simulink model "NetworkModelSimpleIntersectionOptimalControl"  (R2018b)
settings: Solver=VariableStepAuto  StartTime=tStart  StopTime=tFinal  FixedStep=0.001  RelTol=1e-3
values from neighbouring files (symbols this model uses):
  Ax = [0 1  0   0 ... (first row only)    [DroneSubsystemModelling.m]
  Ay = [0 1  0   0 ... (first row only)    [DroneSubsystemModelling.m]
  Bx = [0;0;0;b1]    [DroneSubsystemModelling.m]
  By = [0;0;0;b2]    [DroneSubsystemModelling.m]
  ConflictDrone2andDrone4 = ControlDetectionFunction(tout,PositionXDrone2, PositionYDrone2, PositionXDrone4, PositionYDrone4, ConflictDrone2andDrone4)    [ConflictDetection.m]    (also in ConflictDetectionTEST.m = ControlDetectionFunction(tout,PositionXDrone2TEST, PositionY)
  Cpx = [1 0 0 0]    [DroneSubsystemModelling.m]
  Cpy = [1 0 0 0]    [DroneSubsystemModelling.m]
  Cvx = [0 1 0 0]    [DroneSubsystemModelling.m]
  Cvy = [0 1 0 0]    [DroneSubsystemModelling.m]
  theta2 = -3*180/4    (= -135)    [MotionModelling.m]
  theta4 = -180/4    (= -45)    [MotionModelling.m]
  VelocityStarX2 = vx20    [MotionModelling.m]
  VelocityStarX4 = vx40    [MotionModelling.m]
  VelocityStarY2 = vy20    [MotionModelling.m]
  VelocityStarY4 = vy40    [MotionModelling.m]
  X20 = [x20 vx20 0 0]'    [MotionModelling.m]
  X40 = [x40 vx40 0 0]'    [MotionModelling.m]
  Y20 = [y20 vy20 0 0]'    [MotionModelling.m]
  Y40 = [y40 vy40 0 0]'    [MotionModelling.m]
libraries: simulink x8
settings Model: Creator=CowUser  LastModifiedBy=CowUser

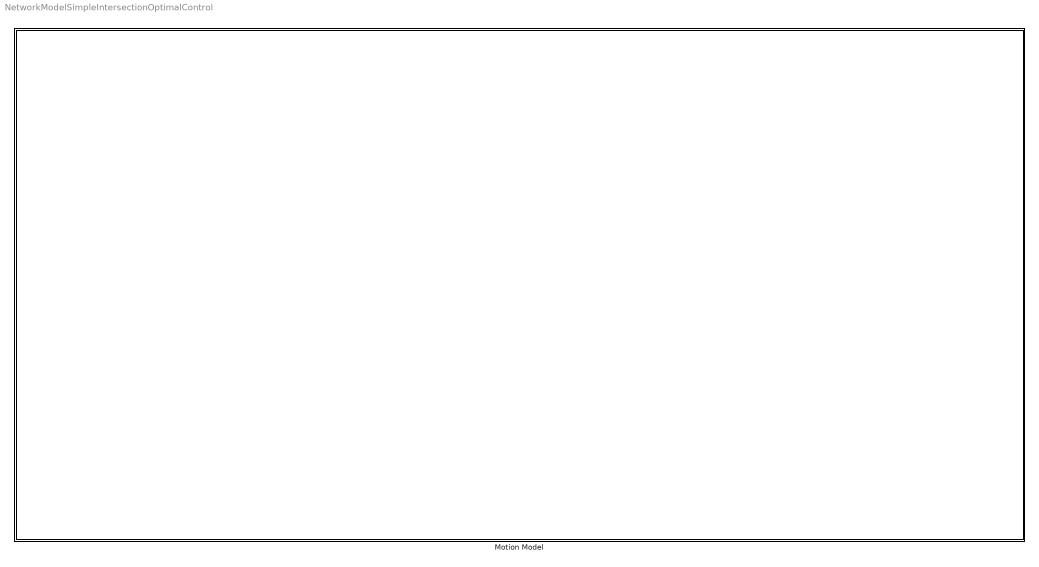
== system NetworkModelSimpleIntersectionOptimalControl ==
  Motion Model : Subsystem

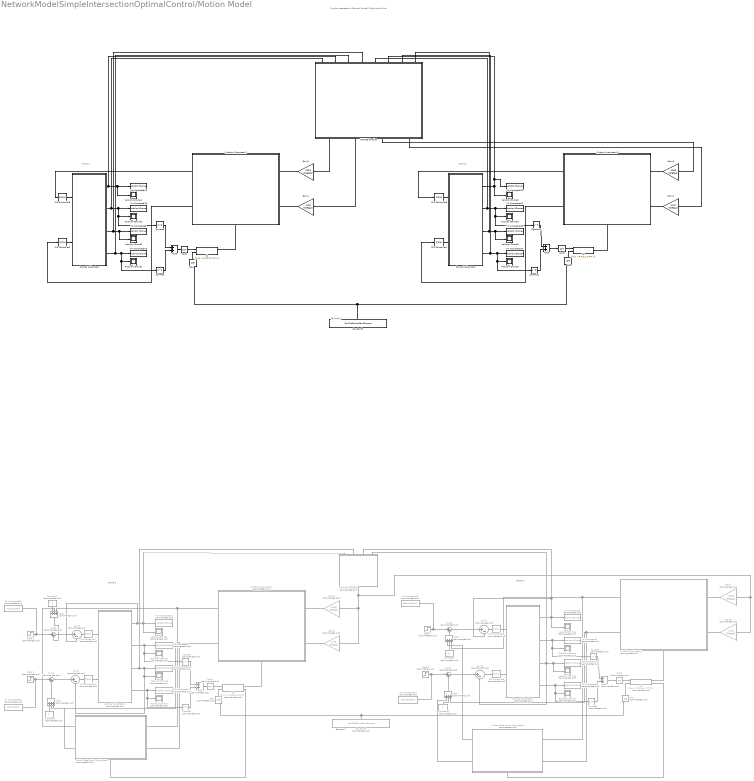
== system NetworkModelSimpleIntersectionOptimalControl/Motion Model ==
  note: Drone j
  note: Drone i
  note: Sample 1
  note: Simple Intersection
      | (Optimal Control)
      |
      | Right Hand Rule
  note: Drone 2
  note: Drone 4
  note: Sample 1
  Add{1..4} (4 alike) : Sum  Commented=on  Inputs=+++
  Add5 : Sum  Commented=on
  Add6 : Sum  Commented=on
  Add8 : Sum
  Add9 : Sum
  Constant{1..4} (4 alike) : Constant  Commented=on  Value=0
  Constant5 : Constant  Commented=on  Value=ConflictDrone2andDrone4
  Constant9 : Constant  Value=ConflictDrone2andDrone4
  Drone2 Subsystem : Subsystem
  Drone2 Subsystem1 : Subsystem  Commented=on
  Drone4 Subsystem : Subsystem
  Drone4 Subsystem1 : Subsystem  Commented=on
  Gain1 : Gain  Gain=sind (theta4)
  Gain2 : Gain  Gain=cosd (theta2)
  Gain3 : Gain  Gain=cosd (theta4)
  Gain4 : Gain  Gain=sind (theta2)
  Gain5 : Gain  Commented=on  Gain=-sind (theta4)
  Gain6 : Gain  Commented=on  Gain=cosd (theta2)
  Gain7 : Gain  Commented=on  Gain=-cosd (theta4)
  Gain8 : Gain  Commented=on  Gain=sind (theta2)
  If Action Subsystem1 : Subsystem  Commented=on  TreatAsAtomicUnit=on
  If Action Subsystem2 : Subsystem  TreatAsAtomicUnit=on
  If Action Subsystem3 : Subsystem  TreatAsAtomicUnit=on
  If Action Subsystem4 : Subsystem  Commented=on  TreatAsAtomicUnit=on
  If1 : If  Commented=on  NumInputs=2  IfExpression=(u1 <= R)&(u2 == 1)  ElseIfExpressions=(u1 > R)&(u2 == 1)  ShowElse=off
  If2 : If  NumInputs=2  IfExpression=(u1 <= R)&(u2 == 1)  ShowElse=off
  If3 : If  Commented=on  NumInputs=2  IfExpression=(u1 <= R)&(u2 == 1)  ElseIfExpressions=(u1 > R)&(u2 == 1)  ShowElse=off
  If4 : If  NumInputs=2  IfExpression=(u1 <= R)&(u2 == 1)  ElseIfExpressions=(u1 > R)&(u2 == 1)  ShowElse=off
  MATLAB Function : MATLAB Function  TreatAsAtomicUnit=on
  MATLAB Function1 : MATLAB Function  Commented=on  TreatAsAtomicUnit=on
  OR1 : Logic  Commented=on  Operator=OR  Inputs=3  IconShape=distinctive  AllPortsSameDT=off  OutDataTypeStr='double'
  OR2 : Logic  Commented=on  Operator=OR  Inputs=3  IconShape=distinctive  AllPortsSameDT=off  OutDataTypeStr='double'
  OR3 : Logic  Operator=OR  Inputs=3  IconShape=distinctive  AllPortsSameDT=off  OutDataTypeStr='double'
  OR4 : Logic  Operator=OR  Inputs=3  IconShape=distinctive  AllPortsSameDT=off  OutDataTypeStr='double'
  PID Controller{1,3,6..7} (4 alike) : simulink/Continuous/PID Controller  Commented=on  Controller=PID  Form=Parallel  TimeDomain=Continuous-time  SampleTime=-1  IntegratorMethod=Forward Euler  FilterMethod=Forward Euler  ControllerParametersSource=internal  P=1.97139727738968e-05  I=1.5233344900537e-08  D=0.00566857635684116  UseFilter=on  N=15.1370363747334  TunerSelectOption=Transfer Function Based (PID Tuner App)  InitialConditionSource=internal  InitialConditionForIntegrator=0  InitialConditionForFilter=0  DifferentiatorICPrevScaledInput=0  ExternalReset=none  TrackingMode=off  Kt=1  LimitOutput=off  UpperSaturationLimit=inf  LowerSaturationLimit=-inf  LinearizeAsGain=on  AntiWindupMode=none  Kb=1  POutMin=[]  POutMax=[]  IOutMin=[]  IOutMax=[]  DOutMin=[]  DOutMax=[]  NOutMin=[]  NOutMax=[]  SumOutMin=[]  SumOutMax=[]  SaturationOutMin=[]  SaturationOutMax=[]  PParamMin=[]  PParamMax=[]  IParamMin=[]  IParamMax=[]  DParamMin=[]  DParamMax=[]  NParamMin=[]  NParamMax=[]  KbParamMin=[]  KbParamMax=[]  KtParamMin=[]  KtParamMax=[]  KbOutMin=[]  KbOutMax=[]  KtOutMin=[]  KtOutMax=[]  IntegratorOutMin=[]  IntegratorOutMax=[]  FilterOutMin=[]  FilterOutMax=[]  SumI1OutMin=[]  SumI1OutMax=[]  SumI2OutMin=[]  SumI2OutMax=[]  SumI3OutMin=[]  SumI3OutMax=[]  SumI4OutMin=[]  SumI4OutMax=[]  SumDOutMin=[]  SumDOutMax=[]  DifferentiatorOutMin=[]  DifferentiatorOutMax=[]  FilterDiffOutCoefMin=[]  FilterDiffOutCoefMax=[]  ReciprocalOutMin=[]  ReciprocalOutMax=[]  SumDenOutMin=[]  SumDenOutMax=[]  SumNumOutMin=[]  SumNumOutMax=[]  DivideOutMin=[]  DivideOutMax=[]  IntegratorContinuousStateAttributes=''  IntegratorStateMustResolveToSignalObject=off  IntegratorRTWStateStorageClass=Auto  FilterContinuousStateAttributes=''  FilterStateMustResolveToSignalObject=off  FilterRTWStateStorageClass=Auto  ParallelPVariant=InternalParameters  IdealPVariant=Disabled  IVariant=InternalParameters  DVariant=InternalParameters  IntegratorVariant=Continuous  SatVariant=Disabled  AWVariant=Passthrough  PCopyVariant=Disabled  TRVariant=Disabled  FdbkBlocksVariant=Forward  IdealPFdbkVariant=Disabled  SatFdbkVariant=Disabled  DerivativeFilterVariant=ContFilter  NVariant=InternalParameters  NCopyVariant=Disabled  FilterICVariant=InternalICsFilter  IntegratorICVariant=InternalICs  ExternalResetVariant=Disabled  TRSumVariant=Passthrough  SumFdbkVariant=Disabled  SumVariant=Sum_PID
  PID Controller{2,4..5,8} (4 alike) : simulink/Continuous/PID Controller  Controller=PID  Form=Parallel  TimeDomain=Continuous-time  SampleTime=-1  IntegratorMethod=Forward Euler  FilterMethod=Forward Euler  ControllerParametersSource=internal  P=1.97139727738968e-05  I=1.5233344900537e-08  D=0.00566857635684116  UseFilter=on  N=15.1370363747334  TunerSelectOption=Transfer Function Based (PID Tuner App)  InitialConditionSource=internal  InitialConditionForIntegrator=0  InitialConditionForFilter=0  DifferentiatorICPrevScaledInput=0  ExternalReset=none  TrackingMode=off  Kt=1  LimitOutput=off  UpperSaturationLimit=inf  LowerSaturationLimit=-inf  LinearizeAsGain=on  AntiWindupMode=none  Kb=1  POutMin=[]  POutMax=[]  IOutMin=[]  IOutMax=[]  DOutMin=[]  DOutMax=[]  NOutMin=[]  NOutMax=[]  SumOutMin=[]  SumOutMax=[]  SaturationOutMin=[]  SaturationOutMax=[]  PParamMin=[]  PParamMax=[]  IParamMin=[]  IParamMax=[]  DParamMin=[]  DParamMax=[]  NParamMin=[]  NParamMax=[]  KbParamMin=[]  KbParamMax=[]  KtParamMin=[]  KtParamMax=[]  KbOutMin=[]  KbOutMax=[]  KtOutMin=[]  KtOutMax=[]  IntegratorOutMin=[]  IntegratorOutMax=[]  FilterOutMin=[]  FilterOutMax=[]  SumI1OutMin=[]  SumI1OutMax=[]  SumI2OutMin=[]  SumI2OutMax=[]  SumI3OutMin=[]  SumI3OutMax=[]  SumI4OutMin=[]  SumI4OutMax=[]  SumDOutMin=[]  SumDOutMax=[]  DifferentiatorOutMin=[]  DifferentiatorOutMax=[]  FilterDiffOutCoefMin=[]  FilterDiffOutCoefMax=[]  ReciprocalOutMin=[]  ReciprocalOutMax=[]  SumDenOutMin=[]  SumDenOutMax=[]  SumNumOutMin=[]  SumNumOutMax=[]  DivideOutMin=[]  DivideOutMax=[]  IntegratorContinuousStateAttributes=''  IntegratorStateMustResolveToSignalObject=off  IntegratorRTWStateStorageClass=Auto  FilterContinuousStateAttributes=''  FilterStateMustResolveToSignalObject=off  FilterRTWStateStorageClass=Auto  ParallelPVariant=InternalParameters  IdealPVariant=Disabled  IVariant=InternalParameters  DVariant=InternalParameters  IntegratorVariant=Continuous  SatVariant=Disabled  AWVariant=Passthrough  PCopyVariant=Disabled  TRVariant=Disabled  FdbkBlocksVariant=Forward  IdealPFdbkVariant=Disabled  SatFdbkVariant=Disabled  DerivativeFilterVariant=ContFilter  NVariant=InternalParameters  NCopyVariant=Disabled  FilterICVariant=InternalICsFilter  IntegratorICVariant=InternalICs  ExternalResetVariant=Disabled  TRSumVariant=Passthrough  SumFdbkVariant=Disabled  SumVariant=Sum_PID
  PositionXDrone1 : Scope
  PositionXDrone2 : Scope  Commented=on
  PositionXDrone3 : Scope
  PositionXDrone4 : Scope  Commented=on
  PositionYDrone1 : Scope
  PositionYDrone2 : Scope  Commented=on
  PositionYDrone3 : Scope
  PositionYDrone4 : Scope  Commented=on
  Sqrt1 : Sqrt  Commented=on  SaturateOnIntegerOverflow=on
  Sqrt2 : Sqrt  Commented=on  SaturateOnIntegerOverflow=on
  Sqrt4 : Sqrt  SaturateOnIntegerOverflow=on
  Sqrt5 : Sqrt  SaturateOnIntegerOverflow=on
  Square{1..4} (4 alike) : Math  Commented=on  Operator=square  SaturateOnIntegerOverflow=on
  Square{8..11} (4 alike) : Math  Operator=square  SaturateOnIntegerOverflow=on
  Step 1 : Step  Commented=on  Time=0  After=VelocityStarX2  SampleTime=0
  Step 2 : Step  Commented=on  Time=0  After=VelocityStarY2  SampleTime=0
  Step 7 : Step  Commented=on  Time=0  After=VelocityStarX4  SampleTime=0
  Step 8 : Step  Commented=on  Time=0  After=VelocityStarY4  SampleTime=0
  Sum{1..8} (8 alike) : Sum  Commented=on  Inputs=|+-
  Switch Case Action Subsystem2 : Subsystem  Commented=on  TreatAsAtomicUnit=on
  Switch Case Action Subsystem3 : Subsystem  Commented=on  TreatAsAtomicUnit=on
  To Workspace1 : ToWorkspace  Commented=on  VariableName=VelocityYDrone  SampleTime=-1
  To Workspace10 : ToWorkspace  VariableName=VelocityYDrone4  SampleTime=-1
  To Workspace11 : ToWorkspace  VariableName=PositionXDrone4  SampleTime=-1
  To Workspace12 : ToWorkspace  VariableName=VelocityXDrone4  SampleTime=-1
  To Workspace14 : ToWorkspace  VariableName=PositionYDrone4  SampleTime=-1
  To Workspace15 : ToWorkspace  VariableName=PositionXDrone2  SampleTime=-1
  To Workspace16 : ToWorkspace  VariableName=VelocityXDrone2  SampleTime=-1
  To Workspace18 : ToWorkspace  VariableName=PositionYDrone2  SampleTime=-1
  To Workspace19 : ToWorkspace  Commented=on  VariableName=VelocityXDrone  SampleTime=-1
  To Workspace2 : ToWorkspace  Commented=on  VariableName=PositionXDrone  SampleTime=-1
  To Workspace20 : ToWorkspace  Commented=on  VariableName=VelocityStarX  SampleTime=-1
  To Workspace21 : ToWorkspace  Commented=on  VariableName=PositionYDrone  SampleTime=-1
  To Workspace22 : ToWorkspace  Commented=on  VariableName=VelocityStarY  SampleTime=-1
  To Workspace23 : ToWorkspace  Commented=on  VariableName=VelocityStarY1  SampleTime=-1
  To Workspace24 : ToWorkspace  Commented=on  VariableName=VelocityYDrone1  SampleTime=-1
  To Workspace3 : ToWorkspace  Commented=on  VariableName=VelocityXDrone1  SampleTime=-1
  To Workspace4 : ToWorkspace  Commented=on  VariableName=VelocityStarX1  SampleTime=-1
  To Workspace5 : ToWorkspace  Commented=on  VariableName=PositionYDrone1  SampleTime=-1
  To Workspace6 : ToWorkspace  Commented=on  VariableName=PositionXDrone1  SampleTime=-1
  To Workspace9 : ToWorkspace  VariableName=VelocityYDrone2  SampleTime=-1
  VelocityXDrone1 : Scope
  VelocityXDrone2 : Scope  Commented=on
  VelocityXDrone3 : Scope
  VelocityXDrone4 : Scope  Commented=on
  VelocityYDrone1 : Scope
  VelocityYDrone2 : Scope  Commented=on
  VelocityYDrone3 : Scope
  VelocityYDrone4 : Scope  Commented=on
  wires:
  Square10/1 -> Add9/1
  PID Controller2/1 -> Drone2 Subsystem/2("InputForceY* ")
  Sqrt4/1 -> If4/1
  If Action Subsystem2/1(dVx2) -> PID Controller8/1
  Gain2/1 -> If Action Subsystem2/1(deltaVx2)
  Constant9/1 -> OR4/3, OR3/1
  Drone2 Subsystem/3(Vy) -> MATLAB Function/4(qDotyi), To Workspace9/1, VelocityYDrone1/1
  Sqrt5/1 -> If2/1
  If Action Subsystem3/1(dVx4) -> PID Controller5/1
  If Action Subsystem3/2(dVy4) -> PID Controller4/1
  PID Controller5/1 -> Drone4 Subsystem/1(InputForceX*)
  If4/1 -> If Action Subsystem2/Action
  Gain3/1 -> If Action Subsystem3/1(deltaVx4)
  Gain4/1 -> If Action Subsystem2/2(deltaVy2)
  OR4/1 -> If4/2
  Drone4 Subsystem/4(y) -> Square11/1, PositionYDrone3/1, To Workspace14/1, MATLAB Function/7(qyj)
  Square9/1 -> Add8/2
  Square8/1 -> Add8/1
  Add9/1 -> Sqrt5/1
  Square11/1 -> Add9/2
  If2/1 -> If Action Subsystem3/Action
  If Action Subsystem2/2(dVy2) -> PID Controller2/1
  PID Controller8/1 -> Drone2 Subsystem/1(InputForceX*)
  OR3/1 -> If2/2
  Drone4 Subsystem/2(x) -> Square10/1, PositionXDrone3/1, To Workspace11/1, MATLAB Function/5(qxj)
  Gain1/1 -> If Action Subsystem3/2(deltaVy4)
  Add8/1 -> Sqrt4/1
  Drone2 Subsystem/2(x) -> MATLAB Function/1(qxi), Square8/1, PositionXDrone1/1, To Workspace15/1
  Drone4 Subsystem/1(Vx) -> MATLAB Function/6(qDotxj), To Workspace12/1, VelocityXDrone3/1
  Drone2 Subsystem/4(y) -> MATLAB Function/3(qyi), To Workspace18/1, Square9/1, PositionYDrone1/1
  PID Controller4/1 -> Drone4 Subsystem/2("InputForceY* ")
  Drone4 Subsystem/3(Vy) -> MATLAB Function/8(qDotyj), VelocityYDrone3/1, To Workspace10/1
  Drone2 Subsystem/1(Vx) -> To Workspace16/1, VelocityXDrone1/1, MATLAB Function/2(qDotxi)
  MATLAB Function1/1(y) -> Gain8/1, Gain6/1, Gain7/1, Gain5/1
  Square3/1 -> Add5/1
  Square2/1 -> Add6/2
  Sum6/1 -> Sum4/1
  Drone4 Subsystem1/3(Vy) -> MATLAB Function1/4(qDotyj), Sum5/2, VelocityYDrone4/1, To Workspace1/1
  Step 7/1 -> Sum6/1, To Workspace4/1
  PID Controller6/1 -> Drone4 Subsystem1/1(InputForceX*)
  Drone4 Subsystem1/1(Vx) -> MATLAB Function1/3(qDotyi), Sum4/2, To Workspace3/1, VelocityXDrone4/1
  Switch Case Action Subsystem3/1(dVx4) -> Add3/1
  If1/1 -> If Action Subsystem4/Action
  Drone2 Subsystem1/4(y) -> To Workspace21/1, Square4/1, PositionYDrone2/1
  Sum3/1 -> PID Controller7/1
  Step 1/1 -> Sum8/1, To Workspace20/1
  Add3/1 -> Sum6/2
  Constant5/1 -> OR2/3, OR1/1
  Drone2 Subsystem1/2(x) -> Square3/1, PositionXDrone2/1, To Workspace6/1
  Drone4 Subsystem1/2(x) -> Square1/1, PositionXDrone4/1, To Workspace2/1
  If3/2 -> Switch Case Action Subsystem2/Action
  If Action Subsystem1/1(dVx2) -> Switch Case Action Subsystem2/1(deltaVx2), Add2/3
  Add5/1 -> Sqrt1/1
  OR1/1 -> If1/2
  Sqrt1/1 -> If3/1
  Switch Case Action Subsystem2/1(dVx2) -> Add2/1
  PID Controller1/1 -> Drone2 Subsystem1/2("InputForceY* ")
  If Action Subsystem4/1(dVx4) -> Switch Case Action Subsystem3/1(deltaVx4), Add3/3
  Gain5/1 -> If Action Subsystem4/2(deltaVy4)
  Constant3/1 -> Add3/2
  Add6/1 -> Sqrt2/1
  Square4/1 -> Add5/2
  Switch Case Action Subsystem3/2(dVy4) -> Add4/1
  Sum1/1 -> PID Controller1/1
  Step 2/1 -> Sum2/1, To Workspace22/1
  Sum7/1 -> Sum5/1
  Drone2 Subsystem1/1(Vx) -> Sum3/2, MATLAB Function1/1(qDotxi), VelocityXDrone2/1, To Workspace19/1
  If Action Subsystem1/2(dVy2) -> Add1/2, Switch Case Action Subsystem2/2(deltaVy2)
  Add2/1 -> Sum8/2
  Add1/1 -> Sum2/2
  If3/1 -> If Action Subsystem1/Action
  Drone4 Subsystem1/4(y) -> Square2/1, PositionYDrone4/1, To Workspace5/1
  Add4/1 -> Sum7/2
  Drone2 Subsystem1/3(Vy) -> To Workspace24/1, Sum1/2, VelocityYDrone2/1, MATLAB Function1/2(qDotxj)
  PID Controller3/1 -> Drone4 Subsystem1/2("InputForceY* ")
  Gain7/1 -> If Action Subsystem4/1(deltaVx4)
  OR2/1 -> If3/2
  Gain8/1 -> If Action Subsystem1/2(deltaVy2)
  Constant2/1 -> Add1/1
  Constant1/1 -> Add2/2
  If1/2 -> Switch Case Action Subsystem3/Action
  Sum5/1 -> PID Controller3/1
  Sum2/1 -> Sum1/1
  Square1/1 -> Add6/1
  Step 8/1 -> To Workspace23/1, Sum7/1
  Sqrt2/1 -> If1/1
  If Action Subsystem4/2(dVy4) -> Switch Case Action Subsystem3/2(deltaVy4), Add4/3
  Sum4/1 -> PID Controller6/1
  Constant4/1 -> Add4/2
  Switch Case Action Subsystem2/2(dVy2) -> Add1/3
  Sum8/1 -> Sum3/1
  PID Controller7/1 -> Drone2 Subsystem1/1(InputForceX*)
  Gain6/1 -> If Action Subsystem1/1(deltaVx2)
  MATLAB Function/1(xDoti_ref) -> Gain2/1
  MATLAB Function/2(yDoti_ref) -> Gain4/1
  MATLAB Function/3(xDotj_ref) -> Gain3/1
  MATLAB Function/4(yDotj_ref) -> Gain1/1

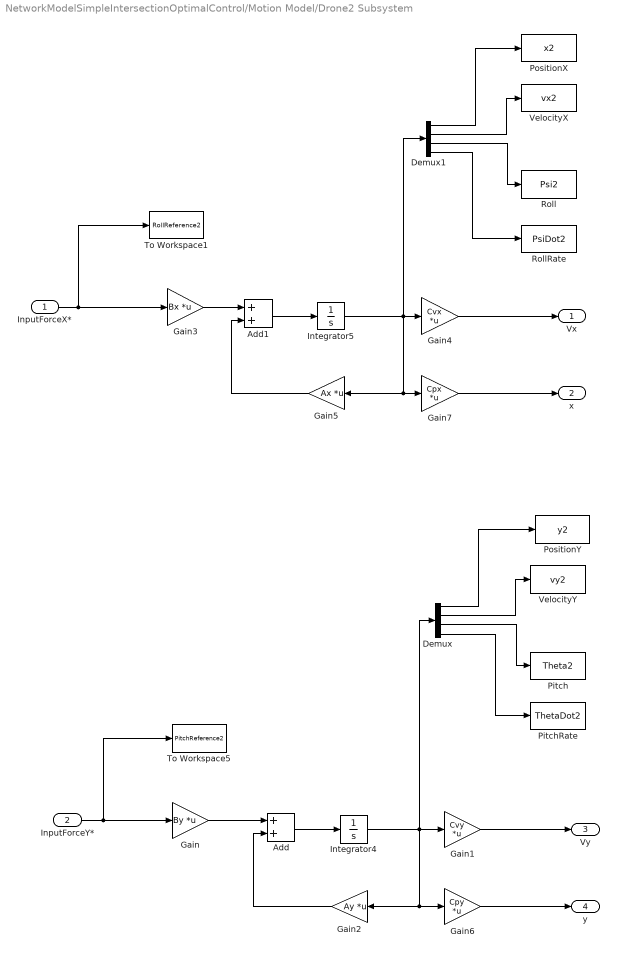
== system NetworkModelSimpleIntersectionOptimalControl/Motion Model/Drone2 Subsystem ==
  InputForceX* : Inport
  "InputForceY* " : Inport  Port=2
  Add : Sum
  Add1 : Sum
  Demux : Demux
  Demux1 : Demux
  Gain : Gain  Gain=By  Multiplication=Matrix(K*u)
  Gain1 : Gain  Gain=Cvy  Multiplication=Matrix(K*u)
  Gain2 : Gain  Gain=Ay  Multiplication=Matrix(K*u)
  Gain3 : Gain  Gain=Bx  Multiplication=Matrix(K*u)
  Gain4 : Gain  Gain=Cvx  Multiplication=Matrix(K*u)
  Gain5 : Gain  Gain=Ax  Multiplication=Matrix(K*u)
  Gain6 : Gain  Gain=Cpy  Multiplication=Matrix(K*u)
  Gain7 : Gain  Gain=Cpx  Multiplication=Matrix(K*u)
  Integrator4 : Integrator  InitialCondition=Y20
  Integrator5 : Integrator  InitialCondition=X20
  Pitch : ToWorkspace  VariableName=Theta2  SampleTime=-1
  PitchRate : ToWorkspace  VariableName=ThetaDot2  SampleTime=-1
  PositionX : ToWorkspace  VariableName=x2  SampleTime=-1
  PositionY : ToWorkspace  VariableName=y2  SampleTime=-1
  Roll : ToWorkspace  VariableName=Psi2  SampleTime=-1
  RollRate : ToWorkspace  VariableName=PsiDot2  SampleTime=-1
  To Workspace1 : ToWorkspace  VariableName=RollReference2  SampleTime=-1
  To Workspace5 : ToWorkspace  VariableName=PitchReference2  SampleTime=-1
  VelocityX : ToWorkspace  VariableName=vx2  SampleTime=-1
  VelocityY : ToWorkspace  VariableName=vy2  SampleTime=-1
  Vx : Outport
  x : Outport  Port=2
  Vy : Outport  Port=3
  y : Outport  Port=4
  wires:
  Demux/1 -> PositionY/1
  Demux1/2 -> VelocityX/1
  Demux1/4 -> RollRate/1
  Demux1/3 -> Roll/1
  Gain4/1 -> Vx/1
  "InputForceY* "/1 -> Gain/1, To Workspace5/1
  Gain/1 -> Add/1
  Demux/4 -> PitchRate/1
  Demux/3 -> Pitch/1
  Add/1 -> Integrator4/1
  Demux1/1 -> PositionX/1
  Gain1/1 -> Vy/1
  InputForceX*/1 -> Gain3/1, To Workspace1/1
  Gain7/1 -> x/1
  Integrator4/1 -> Gain6/1, Gain2/1, Demux/1, Gain1/1
  Demux/2 -> VelocityY/1
  Gain6/1 -> y/1
  Gain3/1 -> Add1/1
  Add1/1 -> Integrator5/1
  Gain2/1 -> Add/2
  Integrator5/1 -> Gain4/1, Gain5/1, Gain7/1, Demux1/1
  Gain5/1 -> Add1/2

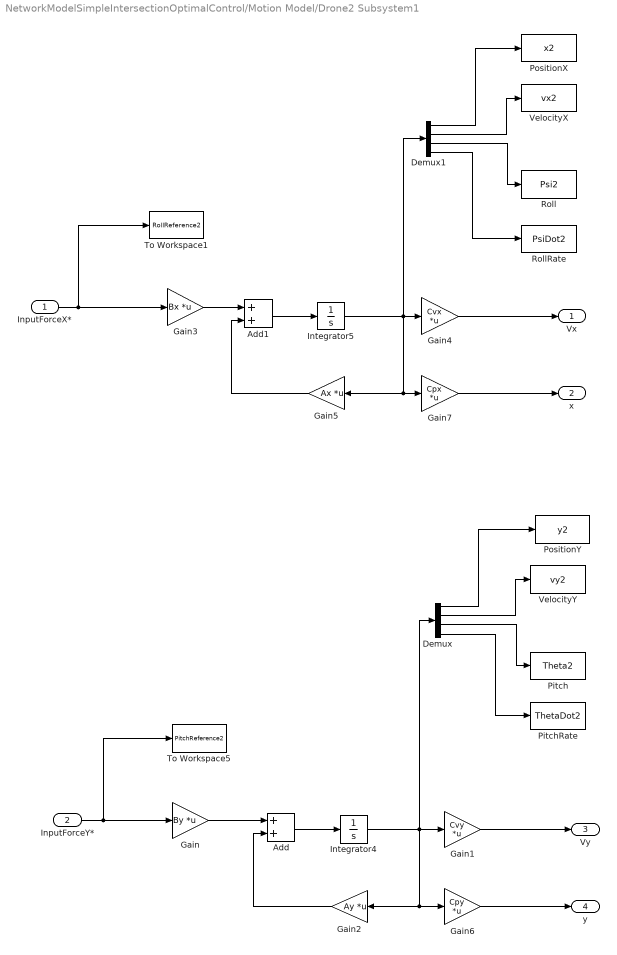
== system NetworkModelSimpleIntersectionOptimalControl/Motion Model/Drone2 Subsystem1 ==
  InputForceX* : Inport
  "InputForceY* " : Inport  Port=2
  Add : Sum
  Add1 : Sum
  Demux : Demux
  Demux1 : Demux
  Gain : Gain  Gain=By  Multiplication=Matrix(K*u)
  Gain1 : Gain  Gain=Cvy  Multiplication=Matrix(K*u)
  Gain2 : Gain  Gain=Ay  Multiplication=Matrix(K*u)
  Gain3 : Gain  Gain=Bx  Multiplication=Matrix(K*u)
  Gain4 : Gain  Gain=Cvx  Multiplication=Matrix(K*u)
  Gain5 : Gain  Gain=Ax  Multiplication=Matrix(K*u)
  Gain6 : Gain  Gain=Cpy  Multiplication=Matrix(K*u)
  Gain7 : Gain  Gain=Cpx  Multiplication=Matrix(K*u)
  Integrator4 : Integrator  InitialCondition=Y20
  Integrator5 : Integrator  InitialCondition=X20
  Pitch : ToWorkspace  VariableName=Theta2  SampleTime=-1
  PitchRate : ToWorkspace  VariableName=ThetaDot2  SampleTime=-1
  PositionX : ToWorkspace  VariableName=x2  SampleTime=-1
  PositionY : ToWorkspace  VariableName=y2  SampleTime=-1
  Roll : ToWorkspace  VariableName=Psi2  SampleTime=-1
  RollRate : ToWorkspace  VariableName=PsiDot2  SampleTime=-1
  To Workspace1 : ToWorkspace  VariableName=RollReference2  SampleTime=-1
  To Workspace5 : ToWorkspace  VariableName=PitchReference2  SampleTime=-1
  VelocityX : ToWorkspace  VariableName=vx2  SampleTime=-1
  VelocityY : ToWorkspace  VariableName=vy2  SampleTime=-1
  Vx : Outport
  x : Outport  Port=2
  Vy : Outport  Port=3
  y : Outport  Port=4
  wires:
  Demux/1 -> PositionY/1
  Demux1/2 -> VelocityX/1
  Demux1/4 -> RollRate/1
  Demux1/3 -> Roll/1
  Gain4/1 -> Vx/1
  "InputForceY* "/1 -> Gain/1, To Workspace5/1
  Gain/1 -> Add/1
  Demux/4 -> PitchRate/1
  Demux/3 -> Pitch/1
  Add/1 -> Integrator4/1
  Demux1/1 -> PositionX/1
  Gain1/1 -> Vy/1
  InputForceX*/1 -> Gain3/1, To Workspace1/1
  Gain7/1 -> x/1
  Integrator4/1 -> Gain6/1, Gain2/1, Demux/1, Gain1/1
  Demux/2 -> VelocityY/1
  Gain6/1 -> y/1
  Gain3/1 -> Add1/1
  Add1/1 -> Integrator5/1
  Gain2/1 -> Add/2
  Integrator5/1 -> Gain4/1, Gain5/1, Gain7/1, Demux1/1
  Gain5/1 -> Add1/2

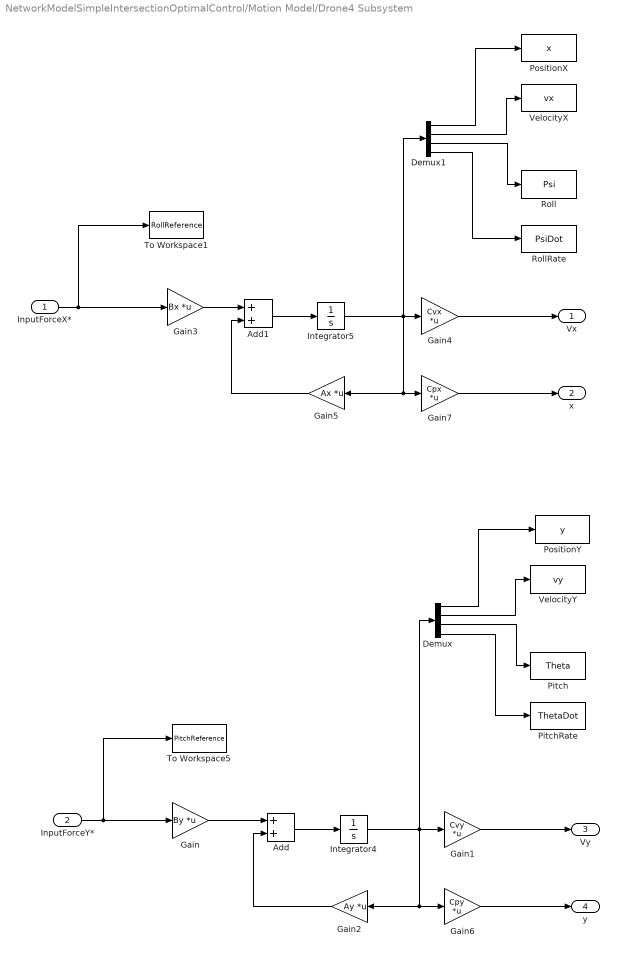
== system NetworkModelSimpleIntersectionOptimalControl/Motion Model/Drone4 Subsystem ==
  InputForceX* : Inport
  "InputForceY* " : Inport  Port=2
  Add : Sum
  Add1 : Sum
  Demux : Demux
  Demux1 : Demux
  Gain : Gain  Gain=By  Multiplication=Matrix(K*u)
  Gain1 : Gain  Gain=Cvy  Multiplication=Matrix(K*u)
  Gain2 : Gain  Gain=Ay  Multiplication=Matrix(K*u)
  Gain3 : Gain  Gain=Bx  Multiplication=Matrix(K*u)
  Gain4 : Gain  Gain=Cvx  Multiplication=Matrix(K*u)
  Gain5 : Gain  Gain=Ax  Multiplication=Matrix(K*u)
  Gain6 : Gain  Gain=Cpy  Multiplication=Matrix(K*u)
  Gain7 : Gain  Gain=Cpx  Multiplication=Matrix(K*u)
  Integrator4 : Integrator  InitialCondition=Y40
  Integrator5 : Integrator  InitialCondition=X40
  Pitch : ToWorkspace  VariableName=Theta  SampleTime=-1
  PitchRate : ToWorkspace  VariableName=ThetaDot  SampleTime=-1
  PositionX : ToWorkspace  VariableName=x  SampleTime=-1
  PositionY : ToWorkspace  VariableName=y  SampleTime=-1
  Roll : ToWorkspace  VariableName=Psi  SampleTime=-1
  RollRate : ToWorkspace  VariableName=PsiDot  SampleTime=-1
  To Workspace1 : ToWorkspace  VariableName=RollReference  SampleTime=-1
  To Workspace5 : ToWorkspace  VariableName=PitchReference  SampleTime=-1
  VelocityX : ToWorkspace  VariableName=vx  SampleTime=-1
  VelocityY : ToWorkspace  VariableName=vy  SampleTime=-1
  Vx : Outport
  x : Outport  Port=2
  Vy : Outport  Port=3
  y : Outport  Port=4
  wires:
  Gain4/1 -> Vx/1
  Demux/2 -> VelocityY/1
  Demux/4 -> PitchRate/1
  Gain3/1 -> Add1/1
  InputForceX*/1 -> Gain3/1, To Workspace1/1
  Gain2/1 -> Add/2
  Demux1/3 -> Roll/1
  Gain7/1 -> x/1
  Add1/1 -> Integrator5/1
  Demux/3 -> Pitch/1
  Gain5/1 -> Add1/2
  Gain6/1 -> y/1
  Integrator5/1 -> Gain4/1, Gain5/1, Gain7/1, Demux1/1
  Gain/1 -> Add/1
  Demux/1 -> PositionY/1
  Add/1 -> Integrator4/1
  Demux1/4 -> RollRate/1
  "InputForceY* "/1 -> Gain/1, To Workspace5/1
  Integrator4/1 -> Gain6/1, Gain2/1, Demux/1, Gain1/1
  Demux1/1 -> PositionX/1
  Demux1/2 -> VelocityX/1
  Gain1/1 -> Vy/1

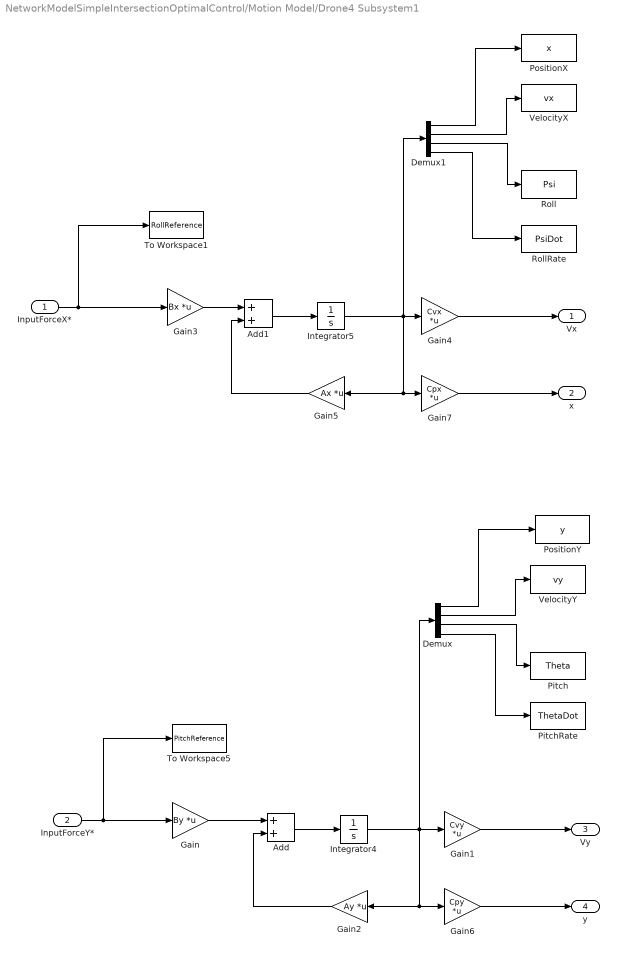
== system NetworkModelSimpleIntersectionOptimalControl/Motion Model/Drone4 Subsystem1 ==
  InputForceX* : Inport
  "InputForceY* " : Inport  Port=2
  Add : Sum
  Add1 : Sum
  Demux : Demux
  Demux1 : Demux
  Gain : Gain  Gain=By  Multiplication=Matrix(K*u)
  Gain1 : Gain  Gain=Cvy  Multiplication=Matrix(K*u)
  Gain2 : Gain  Gain=Ay  Multiplication=Matrix(K*u)
  Gain3 : Gain  Gain=Bx  Multiplication=Matrix(K*u)
  Gain4 : Gain  Gain=Cvx  Multiplication=Matrix(K*u)
  Gain5 : Gain  Gain=Ax  Multiplication=Matrix(K*u)
  Gain6 : Gain  Gain=Cpy  Multiplication=Matrix(K*u)
  Gain7 : Gain  Gain=Cpx  Multiplication=Matrix(K*u)
  Integrator4 : Integrator  InitialCondition=Y40
  Integrator5 : Integrator  InitialCondition=X40
  Pitch : ToWorkspace  VariableName=Theta  SampleTime=-1
  PitchRate : ToWorkspace  VariableName=ThetaDot  SampleTime=-1
  PositionX : ToWorkspace  VariableName=x  SampleTime=-1
  PositionY : ToWorkspace  VariableName=y  SampleTime=-1
  Roll : ToWorkspace  VariableName=Psi  SampleTime=-1
  RollRate : ToWorkspace  VariableName=PsiDot  SampleTime=-1
  To Workspace1 : ToWorkspace  VariableName=RollReference  SampleTime=-1
  To Workspace5 : ToWorkspace  VariableName=PitchReference  SampleTime=-1
  VelocityX : ToWorkspace  VariableName=vx  SampleTime=-1
  VelocityY : ToWorkspace  VariableName=vy  SampleTime=-1
  Vx : Outport
  x : Outport  Port=2
  Vy : Outport  Port=3
  y : Outport  Port=4
  wires:
  Gain4/1 -> Vx/1
  Demux/2 -> VelocityY/1
  Demux/4 -> PitchRate/1
  Gain3/1 -> Add1/1
  InputForceX*/1 -> Gain3/1, To Workspace1/1
  Gain2/1 -> Add/2
  Demux1/3 -> Roll/1
  Gain7/1 -> x/1
  Add1/1 -> Integrator5/1
  Demux/3 -> Pitch/1
  Gain5/1 -> Add1/2
  Gain6/1 -> y/1
  Integrator5/1 -> Gain4/1, Gain5/1, Gain7/1, Demux1/1
  Gain/1 -> Add/1
  Demux/1 -> PositionY/1
  Add/1 -> Integrator4/1
  Demux1/4 -> RollRate/1
  "InputForceY* "/1 -> Gain/1, To Workspace5/1
  Integrator4/1 -> Gain6/1, Gain2/1, Demux/1, Gain1/1
  Demux1/1 -> PositionX/1
  Demux1/2 -> VelocityX/1
  Gain1/1 -> Vy/1

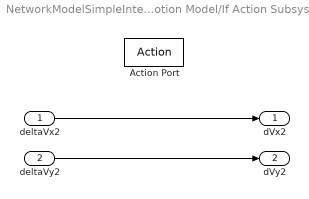
== system NetworkModelSimpleIntersectionOptimalControl/Motion Model/If Action Subsystem1 ==
  deltaVx2 : Inport
  deltaVy2 : Inport  Port=2
  Action Port : ActionPort  ActionType=then
  dVx2 : Outport
  dVy2 : Outport  Port=2
  wires:
  deltaVx2/1 -> dVx2/1
  deltaVy2/1 -> dVy2/1

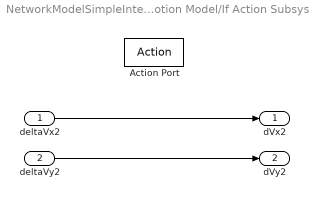
== system NetworkModelSimpleIntersectionOptimalControl/Motion Model/If Action Subsystem2 ==
  deltaVx2 : Inport
  deltaVy2 : Inport  Port=2
  Action Port : ActionPort  ActionType=then
  dVx2 : Outport
  dVy2 : Outport  Port=2
  wires:
  deltaVx2/1 -> dVx2/1
  deltaVy2/1 -> dVy2/1

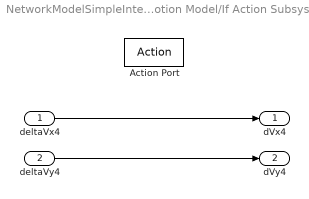
== system NetworkModelSimpleIntersectionOptimalControl/Motion Model/If Action Subsystem3 ==
  deltaVx4 : Inport
  deltaVy4 : Inport  Port=2
  Action Port : ActionPort  ActionType=then
  dVx4 : Outport
  dVy4 : Outport  Port=2
  wires:
  deltaVx4/1 -> dVx4/1
  deltaVy4/1 -> dVy4/1

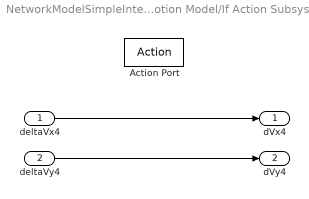
== system NetworkModelSimpleIntersectionOptimalControl/Motion Model/If Action Subsystem4 ==
  deltaVx4 : Inport
  deltaVy4 : Inport  Port=2
  Action Port : ActionPort  ActionType=then
  dVx4 : Outport
  dVy4 : Outport  Port=2
  wires:
  deltaVx4/1 -> dVx4/1
  deltaVy4/1 -> dVy4/1

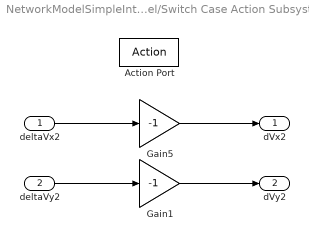
== system NetworkModelSimpleIntersectionOptimalControl/Motion Model/Switch Case Action Subsystem2 ==
  deltaVx2 : Inport
  deltaVy2 : Inport  Port=2
  Action Port : ActionPort  ActionType=elseif
  Gain1 : Gain  Gain=-1
  Gain5 : Gain  Gain=-1
  dVx2 : Outport
  dVy2 : Outport  Port=2
  wires:
  deltaVy2/1 -> Gain1/1
  deltaVx2/1 -> Gain5/1
  Gain5/1 -> dVx2/1
  Gain1/1 -> dVy2/1

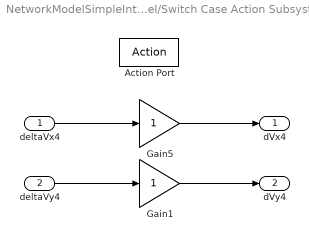
== system NetworkModelSimpleIntersectionOptimalControl/Motion Model/Switch Case Action Subsystem3 ==
  deltaVx4 : Inport
  deltaVy4 : Inport  Port=2
  Action Port : ActionPort  ActionType=elseif
  Gain1 : Gain
  Gain5 : Gain
  dVx4 : Outport
  dVy4 : Outport  Port=2
  wires:
  deltaVy4/1 -> Gain1/1
  deltaVx4/1 -> Gain5/1
  Gain5/1 -> dVx4/1
  Gain1/1 -> dVy4/1

== matlab function NetworkModelSimpleIntersectionOptimalControl/Motion Model/MATLAB Function1 ==
  data: qDotxi input; y output; qDotxj input; qDotyi input; qDotyj input
function y = ClosureRate(qDotxi, qDotxj, qDotyi, qDotyj)

Vmax = 0.2;
K = 1;
Vdiff = K*sqrt((qDotxi - qDotxj)^2 + (qDotyi - qDotyj)^2); 

if abs(Vdiff)>=Vmax/2
    Vdiff = Vmax/2;
end 

y = Vdiff;

== matlab function NetworkModelSimpleIntersectionOptimalControl/Motion Model/MATLAB Function ==
  data: qxi input; qDotxi input; qyi input; qDotyi input; qxj input; qDotxj input; qyj input; xDoti_ref output; qDotyj input; yDoti_ref output; xDotj_ref output; yDotj_ref output
function [xDoti_ref,yDoti_ref,xDotj_ref,yDotj_ref] = OptimalControl(qxi, qDotxi, qyi, qDotyi, qxj, qDotxj, qyj, qDotyj)

Vmax = 0.2;
K = 1;
R = 5;
r = 4;
D = 7;


if (sqrt(qxi^2 + qyi^2) <=  D)&&(sqrt(qxj^2 + qyj^2) <=  D)
    
    p = sqrt((qxi - qxj)^2 + (qyi - qyj)^2); 
    p_dot = sqrt((qDotxi - qDotxj)^2 + (qDotyi - qDotyj)^2); 

    Vj_ref = R*p_dot/p;

    Vi_ref = ((R-r)/(R+r))*R*p_dot/p;


%     if abs(Vi_ref)>= Vmax
%         Vi_ref = Vmax;
%     end 
% 
%     if abs(Vj_ref)>= Vmax
%         Vj_ref = Vmax;
%     end 
    
else 
    
    Vi_ref = Vmax/2;

    Vj_ref = Vmax/2;
    
end        

xDoti_ref = Vi_ref;
yDoti_ref = Vi_ref;
xDotj_ref = Vj_ref;
yDotj_ref = Vj_ref;
